simulink model "vs"  (R2021a)
settings: Solver=VariableStepAuto  StartTime=0.0  StopTime=inf  RelTol=1e-3
undefined symbols (not defined in the file): LF
libraries: instrumentseriallib x3
settings Model: Creator=Sergio  LastModifiedBy=Ravenelco

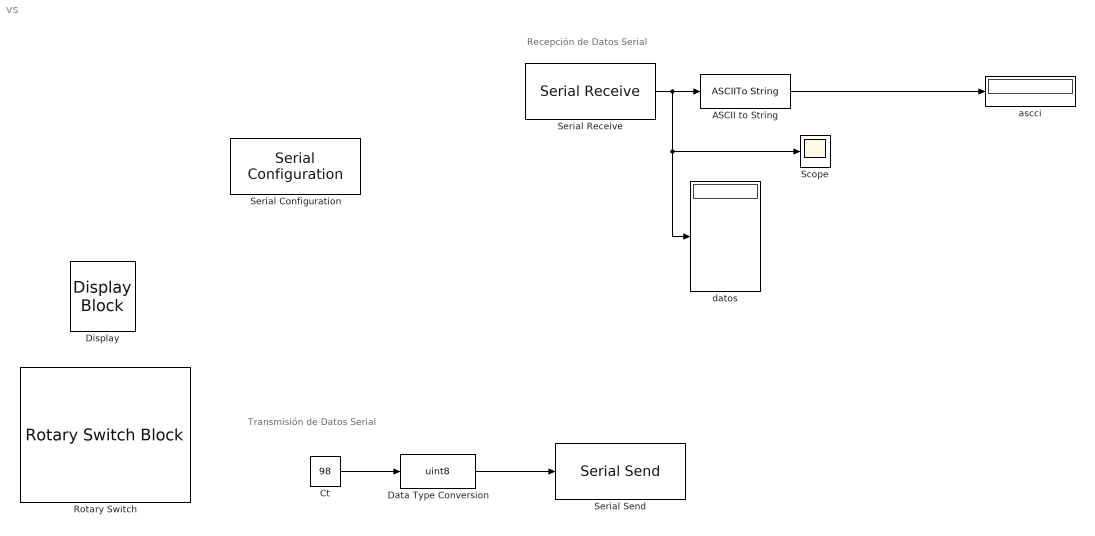
== system vs ==
  note: Transmisión de Datos Serial
  note: Recepción de Datos Serial
  ASCII to String : ASCIIToString
  Ct : Constant  Value=98
  "Data Type Conversion " : DataTypeConversion  OutDataTypeStr=uint8
  Display : DisplayBlock  LabelPosition=Hide  Format=short  Transparency=1  Layout=Fill available space
  Rotary Switch : RotarySwitchBlock
      settings: Values={{'Off', 'Rojo', 'Verde', 'Azul'}, [0 114 103 98]}
  Scope : Scope
  "Serial Configuration " : instrumentseriallib/Serial Configuration  Priority=-200000  Port=COM11  ComPort=COM11  BaudRate=9600  DataBits=8  Parity=none  StopBits=1  ByteOrder=little-endian  FlowControl=none  Timeout=0.01  SimulateUsing=Interpreted execution  BlockInModel=on
  "Serial Receive " : instrumentseriallib/Serial Receive  Priority=1  Port=COM11  ComPort=COM11  DataType=uint8  SaveDataType=uint8  ToggleHeader=off  Header='V'  ToggleTerminator=off  Terminator=LF ('\n')  CustomTerminator=[]  ToggleDataSize=on  DataSize=[1]  EnableBlockingMode=on  ActionDataUnavailable=Output last received value  ActionWhenDataUnavailable=Output last received value  CustomValue=0  SampleTime=0.001  SimulateUsing=Interpreted execution  BlockInModel=on
  "Serial Send " : instrumentseriallib/Serial Send  Priority=1  Port=COM11  ComPort=COM11  Header=[]  Terminator=<none>  CustomTerminator=[]  EnableBlockingMode=on  SimulateUsing=Interpreted execution  BlockInModel=on
  ascci : Display
  datos : Display
  wires:
  "Data Type Conversion "/1 -> "Serial Send "/1
  "Serial Receive "/1 -> Scope/1, datos/1, ASCII to String/1
  ASCII to String/1 -> ascci/1
  Ct/1 -> "Data Type Conversion "/1
